simulink model "aco_ut"  (Simulink 8.1)
settings: Solver=FixedStepDiscrete  StartTime=0.0  StopTime=Inf  FixedStep=0.005  RelTol=1e-3
libraries: siltestlib x3, idiada_lib x3, aco x1
settings Model: Creator=AT015555  LastModifiedBy=AT015555
settings DataIOCC: SignalLoggingSaveFormat=Dataset
settings OptimizationCC: ExpressionDepthLimit=128
settings DebuggingCC: FcnCallInpInsideContextMsg=EnableAllAsError
settings GRTTargetCC: CombineOutputUpdateFcns=on  GRTInterface=off

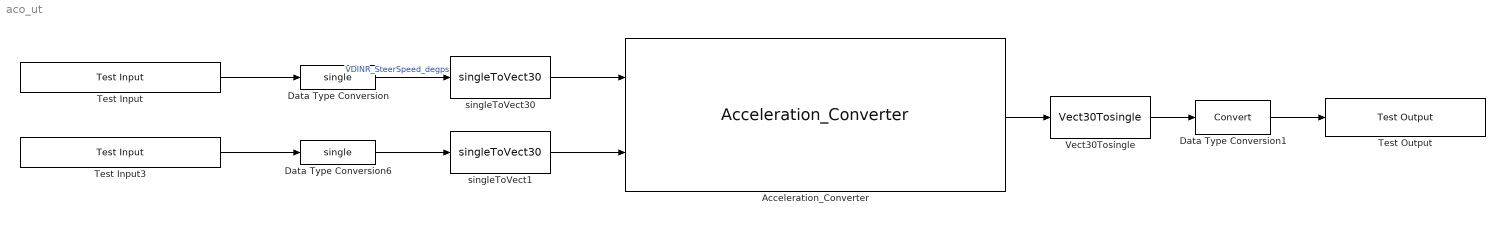
== system aco_ut ==
  Acceleration_Converter : aco/Acceleration_Converter
  Data Type Conversion : DataTypeConversion  OutDataTypeStr=single
  Data Type Conversion1 : DataTypeConversion
  Data Type Conversion6 : DataTypeConversion  OutDataTypeStr=single
  Test Input : siltestlib/Test Input  varname=VPER_TargAccelSingle_mps2  sampletime=0.005
  Test Input3 : siltestlib/Test Input  varname=VPER_TargAttitudeSingle_rad  sampletime=0.005
  Test Output : siltestlib/Test Output  varname=VIFO_TargAccelXVect30_mps2  sampletime=-1
  Vect30Tosingle : idiada_lib/Vect30Tosingle
  singleToVect1 : idiada_lib/singleToVect30
  singleToVect30 : idiada_lib/singleToVect30
  wires:
  Test Input/1 -> Data Type Conversion/1
  Data Type Conversion1/1 -> Test Output/1
  Acceleration_Converter/1 -> Vect30Tosingle/1
  Test Input3/1 -> Data Type Conversion6/1
  Data Type Conversion6/1 -> singleToVect1/1
  Data Type Conversion/1 -> singleToVect30/1  "VDINR_SteerSpeed_degps"
  singleToVect30/1 -> Acceleration_Converter/1
  singleToVect1/1 -> Acceleration_Converter/2
  Vect30Tosingle/1 -> Data Type Conversion1/1
